simulink model "positionctrl_sim"  (Simulink 7.5)
settings: Solver=ode45  StartTime=0.0  StopTime=5  RelTol=1e-3
StopFcn:
  | save_system(vars.simfilename);
CloseFcn:
  | save_system(vars.simfilename); sim(vars.simfilename);vars.simtime = str2num(get_param(vars.simfilename,'StopTime'));set(guiel.hSimtime,'String',num2str(vars.simtime));if strcmp(vars.simfilename(end-2:end),'sim') vars.L= motorParams(1,1); vars.R= motorParams(1,2); vars.J= motorParams(1,3);vars.b= motorParams(1,4); vars.Kb= motorParams(1,5); vars.Km= motorParams(1,6);if (min(size(motorParams)) == 9) vars.P= motorParams(1,7); vars.I= motorParams(1,8); vars.D= motorParams(1,9);else;vars.P= NaN; vars.I= NaN; vars.D= NaN;end;clear motorParams; [vars.numericTF vars.symbolTF] = calcTF2(vars);end,
settings Model: Creator=Dan  LastModifiedBy=Dan
settings DataIOCC: MaxDataPoints=10000
settings OptimizationCC: BlockReduction=off  BooleanDataType=off  InitFltsAndDblsToZero=on
settings DebuggingCC: SaveWithParameterizedLinksMsg=none  SignalResolutionControl=TryResolveAllWithWarning  SolverPrmCheckMsg=none  MultiTaskDSMMsg=warning  MultiTaskCondExecSysMsg=none  StrictBusMsg=None
settings HardwareCC: TargetUnknown=on
settings RTWCC: IncludeERTFirstTime=on
settings GRTTargetCC: TargetFcnLib=ansi_tfl_tmw.mat

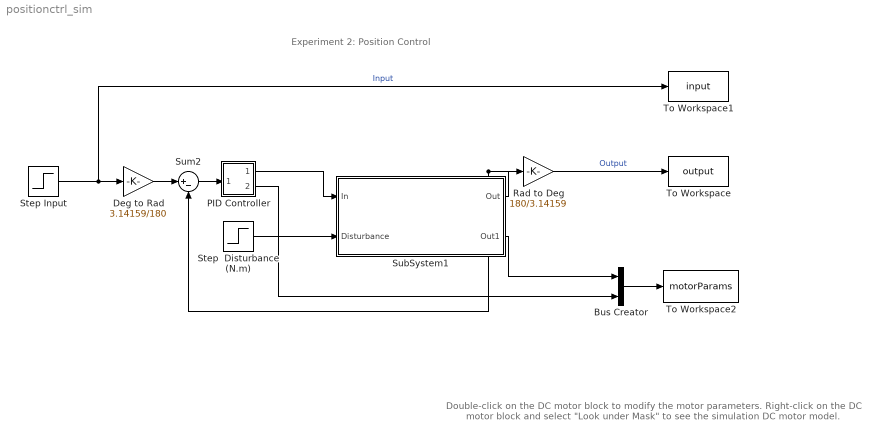
== system positionctrl_sim ==
  note: Experiment 2: Position Control
  note: Double-click on the
      | DC motor block to modify
      | the motor parameters.
      |
      | Right-click on the DC motor
      | block and select "Look under
      | Mask" to see the simulation
      | DC motor model.
  Bus Creator : BusCreator  Inputs=2
  Deg to Rad : Gain  Gain=3.14159/180  ParameterDataType=sfix(16)  ParameterScaling=2^0  OutDataType=sfix(16)  OutScaling=2^0  SaturateOnIntegerOverflow=on  OutDataTypeStr=Inherit: Same as input  ParamDataTypeStr=Inherit: Same as input
  PID Controller : Subsystem  AncestorBlock=simulink_extras/Additional Linear/PID Controller  mask(PID Controller){P=0.9, I=0.4, D=0}
      mask prompts: P "Proportional:"; I "Integral:"; D "Derivative:"
      mask help:
      | Enter expressions for proportional, integral, and derivative terms.
      | P+I/s+Ds
      mask Help: This block implements a PID controller where parameters are entered for the Proportional, Integral and Derivative terms. Unmask this block to see how it works. The derivative term is implemented using a true derivative block.
      mask Display: disp('PID')
  Rad to Deg : Gain  Gain=180/3.14159  ParameterDataType=sfix(16)  ParameterScaling=2^0  OutDataType=sfix(16)  OutScaling=2^0  SaturateOnIntegerOverflow=on  OutDataTypeStr=Inherit: Same as input  ParamDataTypeStr=Inherit: Same as input
  Step  Disturbance (N.m) : Step  Time=0  After=-0.1  SampleTime=0
  Step Input : Step  Time=0  After=160  SampleTime=0
  SubSystem1 : Subsystem  mask{L=0.00056, R=1.35, J=0.0037491, b=0.000792, Kb=0.10, Km=0.10}
      mask prompts: L "Armature Inductance (L [H])"; R "Armature Resistance (R [ohm])"; J "Motor and Load Inertia (J [kg.m^2])"; b "Viscous damping friction (b [kg.m^2/s])"; Kb "Back emf constant (Kb [V/rad/s])"; Km "Motor constant (Km [N.m/A])"
      mask Display: disp('DC Motor (Position Output)')
  Sum2 : Sum  Inputs=|+-  OutDataType=sfix(16)  OutScaling=2^0  SaturateOnIntegerOverflow=on  InputSameDT=on  OutDataTypeStr=Inherit: Same as first input
  To Workspace : ToWorkspace  VariableName=output  SampleTime=-1  SaveFormat=Structure With Time
  To Workspace1 : ToWorkspace  VariableName=input  SampleTime=-1  SaveFormat=Structure With Time
  To Workspace2 : ToWorkspace  VariableName=motorParams  SampleTime=-1  SaveFormat=Array
  wires:
  Rad to Deg/1 -> To Workspace/1  "Output"
  SubSystem1/1(Out) -> Sum2/2, Rad to Deg/1
  Sum2/1 -> PID Controller/1(In_1)
  Deg to Rad/1 -> Sum2/1
  Step Input/1 -> Deg to Rad/1, To Workspace1/1  "Input"
  Step  Disturbance (N.m)/1 -> SubSystem1/2(Disturbance)
  PID Controller/1(Out_1) -> SubSystem1/1(In)
  Bus Creator/1 -> To Workspace2/1
  SubSystem1/2(Out1) -> Bus Creator/1
  PID Controller/2(Parameters) -> Bus Creator/2

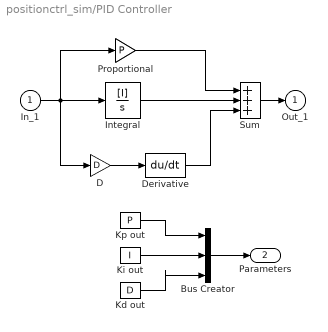
== system positionctrl_sim/PID Controller ==
  In_1 : Inport  OutDataType=sfix(16)  OutScaling=2^0
  Bus Creator : BusCreator  Inputs=3
  D : Gain  Gain=D  ParameterDataType=sfix(16)  ParameterScaling=2^0  OutDataType=sfix(16)  OutScaling=2^0  SaturateOnIntegerOverflow=on  OutDataTypeStr=Inherit: Same as input  ParamDataTypeStr=Inherit: Same as input
  Derivative : Derivative
  Integral : TransferFcn  Numerator=[I]  Denominator=[1 0]
  Kd out : Constant  Value=D  OutDataType=sfix(16)  OutScaling=2^0
  Ki out : Constant  Value=I  OutDataType=sfix(16)  OutScaling=2^0
  Kp out : Constant  Value=P  OutDataType=sfix(16)  OutScaling=2^0
  Proportional : Gain  Gain=P  ParameterDataType=sfix(16)  ParameterScaling=2^0  OutDataType=sfix(16)  OutScaling=2^0  SaturateOnIntegerOverflow=on  OutDataTypeStr=Inherit: Same as input  ParamDataTypeStr=Inherit: Same as input
  Sum : Sum  Inputs=+++  OutDataType=sfix(16)  OutScaling=2^0  SaturateOnIntegerOverflow=on  InputSameDT=on  OutDataTypeStr=Inherit: Same as first input
  Out_1 : Outport  OutDataType=sfix(16)  OutScaling=2^0  InitialOutput=0
  Parameters : Outport  Port=2  OutDataType=sfix(16)  OutScaling=2^0
  wires:
  Proportional/1 -> Sum/1
  Integral/1 -> Sum/2
  Derivative/1 -> Sum/3
  In_1/1 -> Integral/1, Proportional/1, D/1
  Sum/1 -> Out_1/1
  D/1 -> Derivative/1
  Kd out/1 -> Bus Creator/3
  Bus Creator/1 -> Parameters/1
  Kp out/1 -> Bus Creator/1
  Ki out/1 -> Bus Creator/2

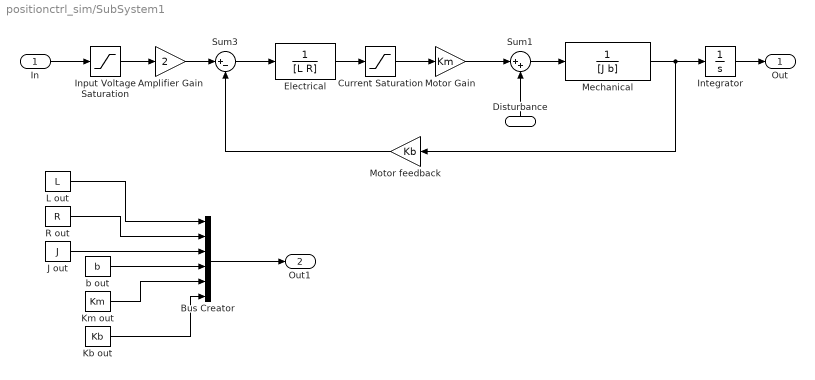
== system positionctrl_sim/SubSystem1 ==
  In : Inport  OutDataType=sfix(16)  OutScaling=2^0
  Disturbance : Inport  Port=2  OutDataType=sfix(16)  OutScaling=2^0
  Amplifier Gain : Gain  Gain=2  ParameterDataType=sfix(16)  ParameterScaling=2^0  OutDataType=sfix(16)  OutScaling=2^0  SaturateOnIntegerOverflow=on  OutDataTypeStr=Inherit: Same as input  ParamDataTypeStr=Inherit: Same as input
  Bus Creator : BusCreator  Inputs=6
  Current Saturation : Saturate  UpperLimit=+4  LowerLimit=-4
  Electrical : TransferFcn  Denominator=[L R]
  Input Voltage Saturation : Saturate  UpperLimit=+10  LowerLimit=-10
  Integrator : Integrator
  J out : Constant  Value=J  OutDataType=sfix(16)  OutScaling=2^0
  Kb out : Constant  Value=Kb  OutDataType=sfix(16)  OutScaling=2^0
  Km out : Constant  Value=Km  OutDataType=sfix(16)  OutScaling=2^0
  L out : Constant  Value=L  OutDataType=sfix(16)  OutScaling=2^0
  Mechanical : TransferFcn  Denominator=[J b]
  Motor Gain : Gain  Gain=Km  ParameterDataType=sfix(16)  ParameterScaling=2^0  OutDataType=sfix(16)  OutScaling=2^0  SaturateOnIntegerOverflow=on  OutDataTypeStr=Inherit: Same as input  ParamDataTypeStr=Inherit: Same as input
  Motor feedback : Gain  Gain=Kb  ParameterDataType=sfix(16)  ParameterScaling=2^0  OutDataType=sfix(16)  OutScaling=2^0  SaturateOnIntegerOverflow=on  OutDataTypeStr=Inherit: Same as input  ParamDataTypeStr=Inherit: Same as input
  R out : Constant  Value=R  OutDataType=sfix(16)  OutScaling=2^0
  Sum1 : Sum  Inputs=|++  OutDataType=sfix(16)  OutScaling=2^0  SaturateOnIntegerOverflow=on  InputSameDT=on  OutDataTypeStr=Inherit: Same as first input
  Sum3 : Sum  Inputs=|+-  OutDataType=sfix(16)  OutScaling=2^0  SaturateOnIntegerOverflow=on  InputSameDT=on  OutDataTypeStr=Inherit: Same as first input
  b out : Constant  Value=b  OutDataType=sfix(16)  OutScaling=2^0
  Out : Outport  OutDataType=sfix(16)  OutScaling=2^0
  Out1 : Outport  Port=2  OutDataType=sfix(16)  OutScaling=2^0
  wires:
  Current Saturation/1 -> Motor Gain/1
  Input Voltage Saturation/1 -> Amplifier Gain/1
  Amplifier Gain/1 -> Sum3/1
  In/1 -> Input Voltage Saturation/1
  Sum3/1 -> Electrical/1
  Mechanical/1 -> Motor feedback/1, Integrator/1
  Electrical/1 -> Current Saturation/1
  Motor feedback/1 -> Sum3/2
  Integrator/1 -> Out/1
  Disturbance/1 -> Sum1/2
  Motor Gain/1 -> Sum1/1
  Sum1/1 -> Mechanical/1
  L out/1 -> Bus Creator/1
  R out/1 -> Bus Creator/2
  J out/1 -> Bus Creator/3
  b out/1 -> Bus Creator/4
  Km out/1 -> Bus Creator/5
  Kb out/1 -> Bus Creator/6
  Bus Creator/1 -> Out1/1
